simulink model "AttitudePlayground"  (R2024b)
settings: Solver=FixedStepAuto  StartTime=0.0  StopTime=inf  FixedStep=delta_t  RelTol=1e-3  EnableMultiTasking=on
values from neighbouring files (symbols this model uses):
  A = [eye(3), delta_t * eye(3) ... (first row only)    [AttitudePlayground_Vars.m]    (also in ParameterIdentification.m = [0 1)
  A_ESO = [1-l1_ESO, delta_t-l1_ESO*delta_t ... (first row only)    [AttitudePlayground_Vars.m]
  A_kalman = [1 delta_t ... (first row only)    [AttitudePlayground_Vars.m]    (also in ControlSystem_Vars.m)
  acc_sigma = 0.2 * calc_sigma(acc_pp)    [AttitudePlayground_Vars.m]    (also in ControlSystem_Vars.m)
  alpha_comp_pitch = calc_alpha(0.1, delta_t)    [AttitudePlayground_Vars.m]
  alpha_comp_roll = calc_alpha(0.1, delta_t)    [AttitudePlayground_Vars.m]
  alpha_comp_yaw = calc_alpha(1, delta_t)    [AttitudePlayground_Vars.m]
  B = zeros(6,3)    [AttitudePlayground_Vars.m]    (also in ParameterIdentification.m = [0)
  b_ESO = [b0_ESO*delta_t - l1_ESO*b0_ESO*delta_t ... (first row only)    [AttitudePlayground_Vars.m]
  bias_0 = [0, 0, 0]    [AttitudePlayground_Vars.m]
  bias_sigma = 0.000000001    (= 1e-09)    [AttitudePlayground_Vars.m]
  C = eye(6)    [AttitudePlayground_Vars.m]    (also in ParameterIdentification.m = [1 0])
  C_kalman = eye(2)    [AttitudePlayground_Vars.m]    (also in ControlSystem_Vars.m)
  delta_t = 0.01    [AttitudePlayground_Vars.m]    (also in ControlSystem_Vars.m; ParameterIdentification.m = t2 - t1)
  gyro_sigma = 1*((pi/180) * (0.07))    (= 0.0012217304764)    [AttitudePlayground_Vars.m]    (also in ControlSystem_Vars.m)
  gyro_sigma_3d = [1*gyro_sigma, 1*gyro_sigma, gyro_sigma]    [AttitudePlayground_Vars.m]    (also in ControlSystem_Vars.m)
  k_i_mahony = 0.0057    [AttitudePlayground_Vars.m]
  k_p_mahony = 0.42    [AttitudePlayground_Vars.m]
  l = [l1_ESO, l2_ESO]'    [AttitudePlayground_Vars.m]
  mag_sigma = 0.8 * calc_sigma(mag_pp)    [AttitudePlayground_Vars.m]
  P_0 = eye(4)    [AttitudePlayground_Vars.m]    (also in ControlSystem_Vars.m)
  P_0_gb = eye(7)    [AttitudePlayground_Vars.m]
  q_init = [cos(initial_yaw/2), 0, 0, sin(initial_yaw/2)]    [AttitudePlayground_Vars.m]
  q_sigma = 0.001    [AttitudePlayground_Vars.m]    (also in ControlSystem_Vars.m)
  R = 1.8 * diag([0.001396263^2, 0.0016580628^2, 0.05^2, ((pi/180) *              (0.05))^2, ((pi/180) * (0.07))^2, ((pi/180) * (0.07))^2])    [AttitudePlayground_Vars.m]    (also in ControlSystem_Vars.m = 0.015625)
  R_kalman = diag([(calc_sigma(0.8))^2, (0.07)^2])    [AttitudePlayground_Vars.m]    (also in ControlSystem_Vars.m)
  r_qekf = 1/sqrt(cos(magnetic_dip_angle_theta)^2 +      sin(magnetic_dip_angle_theta)^2)  * transpose([cos(magnetic_dip_angle_theta),0, sin(magnetic_dip_angle_theta)])    [AttitudePlayground_Vars.m]
  step_time = 10    [AttitudePlayground_Vars.m]
  tau_pitch_comp = 0.5    [AttitudePlayground_Vars.m]
  tau_roll_comp = 0.5    [AttitudePlayground_Vars.m]
  tau_yaw_comp = 3    [AttitudePlayground_Vars.m]
  Ts = delta_t    (= 0.01)    [AttitudePlayground_Vars.m]
  Ts2 = delta_t/2    (= 0.005)    [AttitudePlayground_Vars.m]
  Ts_IMU = delta_t    (= 0.01)    [AttitudePlayground_Vars.m]
  voltage_divider_Vout_max = 1.728    [AttitudePlayground_Vars.m]
undefined symbols (not defined in the file or in its folder): DiscIntNeverNeededParam, Discrete, Newton, Raphson, Time
libraries: simulink_extras x26, dspsigops x5, bbblueActuatorLib x4, ctrlSharedLib x2, matrix_library x2, dspmathops x2, dspstat3 x1, bbblueSensorLib x1, simulink x1, dspfdesign x1, bbblueBasicLib x1, vrlib x1
(part 1 of 3)
settings Model: ExtModeBatchMode=on  ExtModeTrigDuration=100  Creator=Henrik  LastModifiedBy=Henrik
settings SolverCC: PositivePriorityOrder=on
settings OptimizationCC: DefaultParameterBehavior=Inlined  EnhancedBackFolding=on  PassReuseOutputArgsAs=Individual arguments  ZeroExternalMemoryAtStartup=off  ZeroInternalMemoryAtStartup=off  MaxStackSize=64  OptimizeBlockOrder=speed  DifferentSizesBufferReuse=on  OptimizationCustomize=off  EfficientTunableParamExpr=on
settings DebuggingCC: ParameterTunabilityLossMsg=error
settings HardwareCC: ProdBitPerPointer=32  ProdBitPerSizeT=32  ProdBitPerPtrDiffT=32  ProdLargestAtomicInteger=Long  ProdLargestAtomicFloat=Double  ProdWordSize=32  ProdHWDeviceType=ARM Compatible->ARM Cortex-A (32-bit)  UseEmbeddedCoderFeatures=off
settings SFSimCC: MATLABDynamicMemAlloc=off
settings RTWCC: Description=Embedded Coder  SystemTargetFile=ert.tlc  HardwareBoard=BeagleBone Blue  TLCOptions="-aInlineSetEventsForThisBaseRateFcn=TLC_FALSE -aSuppressMultiTaskScheduler=TLC_FALSE  -aRateBasedStepFcn=0"  TemplateMakefile=ert_default_tmf  Toolchain=GNU GCC BeagleBone Blue
settings CodeAppCC: ForceParamTrailComments=on  IgnoreCustomStorageClasses=off  OperatorAnnotations=on  SimulinkDataObjDesc=on  SFDataObjDesc=on  InsertBlockDesc=on
settings ERTTargetCC: SupportNonInlinedSFcns=on  SupportVariableSizeSignals=on

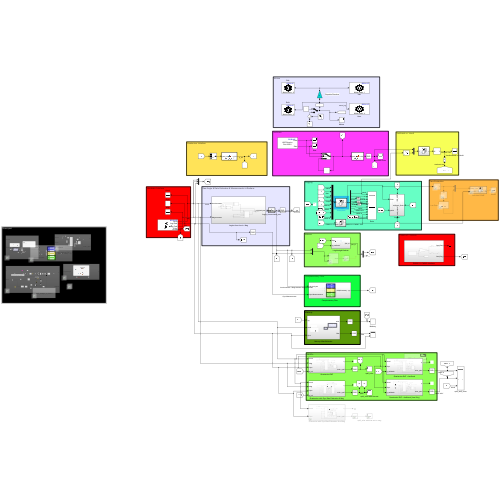
[thumbnail: Simulink's stored preview of the top-level diagram]
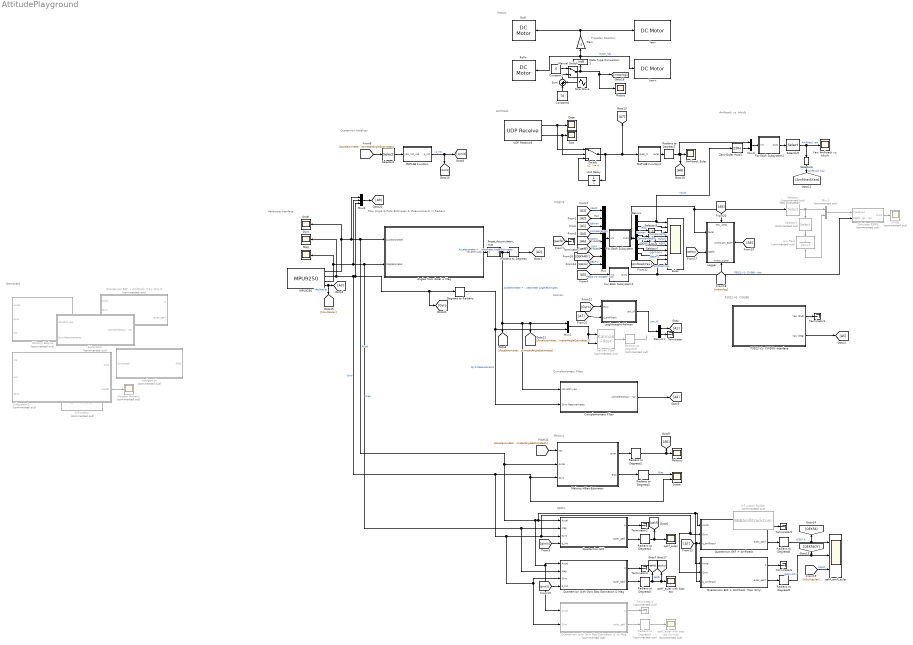
== system AttitudePlayground ==
  note: Graveyard
  note: Propeller Direction
  note: Motors
  note: Quaternion Initializer
  note: Amfitrack vs. Inbuilt
  note: Amfitrack
  note: QEKFs
  note: Mahony
  note: Yaw Evaluation
  note: P3022-V1- CW360
  note: Logging
  note: Kalman
  note: Raw Angle & Rate Estimates & Measurements in Radians
  note: Hardware Interface
  note: Complementary Filter
  Accel : Scope
  Amfitrack Euler : Scope
  Angle_Accumulator_mat : Subsystem  TreatAsAtomicUnit=on
  Angles from Accel + Mag : Subsystem
  Calculate RSME : Subsystem  Commented=on  TreatAsAtomicUnit=on
  Complementary Filter : Subsystem
  Constant1 : Constant  Value=0
  Constant2 : Constant  Value=70
  Data : Scope
  Data Type Conversion1 : DataTypeConversion  OutDataTypeStr=int8  SaturateOnIntegerOverflow=off  RndMeth=Floor
  Degrees to Radians : simulink_extras/Transformations/Degrees to Radians
  Demux : Demux  Outputs=8
  Demux1 : Demux  Outputs=2
  Euler : Scope  NumInputPorts=10
  For Each Subsystem : Subsystem  TreatAsAtomicUnit=on
  For Each Subsystem1 : Subsystem  TreatAsAtomicUnit=on
  For Each Subsystem2 : Subsystem  TreatAsAtomicUnit=on
  Gain : Gain  Gain=-1  OutDataTypeStr=int8
  Gyro : Scope
  Hossein Mahony : Scope  Commented=on
  Kalman Filter : ctrlSharedLib/Kalman Filter  Commented=on  TimeDomain=Discrete-Time  UseCurrentEstimator=on  ModelSource=Individual A, B, C, D matrices  ModelSourceVariable=ss(0.95,1,1,0,1)  A=A  B=B  C=C  D=0  NumberOfStates=1  NumberOfInputs=1  NumberOfOutputs=1  InitialEstimateSource=Input port  X0=0  P0=10  UseK=off  UseGH=off  NumberOfProcessNoiseInputs=1  G=1  TimeInvariantG=on  H=0  TimeInvariantH=on  Q=Q  TimeInvariantQ=on  R=R  TimeInvariantR=on  N=0  TimeInvariantN=on  AddInputPort=off  AddEnablePort=off  OutputEstimatedY=off  OutputP=off  Ts=delta_t
  Leightweight-Kalman : Subsystem
  Logger : Subsystem
      settings: PortSchema="{\"entries\":[{\"content\":{\"sides\":[{\"content\":{\"connectorIds\":[\"In1\",\"In2\"]},\"type\":\"ConnectorPlacement.EquallySpacedRectSide\",\"uuid\":\"65dae65f-b2e3-411c-80c9-991e84581ea0\"},{\"content\":{\"connectorIds\":[\"In5\"],\"side\":\"RIGHT\"},\"type\":\"ConnectorPlacement.EquallySpacedRectSide\",\"uuid\":\"096d2477-2900-49bd-8ed4-d95fcaab5e6a\"},{\"content\":{\"connectorIds\":[\"In3\"],\"side\":\"TOP\"},\"type\":\"ConnectorPlacement.EquallySpacedRectSide\",\"uuid\":\"63021306-1025-463e-9144-c93885efa2cd\"},{\"content\":{\"connectorIds\":[\"In4\"],\"side\":\"BOTTOM\"},\"type\":\"ConnectorPlacement.EquallySpacedRectSide\",\"uuid\":\"f0130dd7-b4e5-4c0e-a86a-26aff2d064e3\"}]},\"type\":\"ConnectorPlacement.EquallySpacedConnector\",\"uuid\":\"57989227-06af-4d59-a161-01dcfc1f7af4\"}],\"packageUris\":[\"http://schema.mathworks.com/mf0/Connector/R2020b\"],\"version\":\"1.0\"}"
  Low Pass : TransferFcn  Commented=on  Denominator=[10 1]
  MATLAB Function : MATLAB Function  TreatAsAtomicUnit=on
  MATLAB Function1 : MATLAB Function  TreatAsAtomicUnit=on
  MPU9250 : bbblueSensorLib/MPU9250  OperationMode=DMP  Accel=on  AngularRate=on  Ak8963Field=on  EulerAngles=on  Quat=off  AccelRange=2G  Acceldlpf=1  GyroRange=250 dps  Gyrodlpf=1  DmpOdr=200 Hz  SampleTime=delta_t
  Mag : Scope
  Mahony : Scope
  Mahony Backup : Subsystem  Commented=on
  Mahony+Bias-Estimator : Subsystem
  Manual Switch : ManualSwitch
  Motors : Scope
  Mux : Mux  Inputs=8
  Mux1 : Mux  Inputs=2
  Mux2 : Mux  Commented=on  Inputs=2
  Mux3 : Mux  Inputs=2
  Mux4 : Mux  Inputs=3
  P3022-V1- CW360 -Interface : Subsystem
  Quarternion EKF : Subsystem
  Quarternion EKF + Amfitrack : Subsystem
  Quarternion EKF + Amfitrack (Yaw Only) : Subsystem
  Quarternion EKF + Amfitrack (Yaw Only)1 : Subsystem  Commented=on
  Quarternion with Gyro Bias Estimation & Mag : Subsystem
  Quarternion with Gyro Bias Estimation & no Mag : Subsystem  Commented=on
  RMSE : Scope  Commented=on
  Radians to Degrees{,2..5,7..9} (8 alike) : simulink_extras/Transformations/Radians to Degrees
  Radians to Degrees1 : simulink_extras/Transformations/Radians to Degrees  Commented=on
  Radians to Degrees6 : simulink_extras/Transformations/Radians to Degrees  Commented=on
  Roll+ : bbblueActuatorLib/DC Motor  index=3  stopaction=Free Spin  SimulateUsing=Code generation
  Roll- : bbblueActuatorLib/DC Motor  index=2  stopaction=Free Spin  SimulateUsing=Code generation
  S-Function : S-Function  Commented=on  FunctionName=amfi_beagle_s_func.c  SFunctionDeploymentMode=off  EnableBusSupport=off
  S-Function Builder : S-Function  Commented=on  FunctionName=BBBAmflitrackCom  SFunctionModules=BBBAmflitrackCom_wrapper.cpp  SFunctionDeploymentMode=off  EnableBusSupport=off  mask(S-Function Builder){}
      mask help: Simulink:masks:SFunctionBuilder_MD
      mask init:
      | val = [[.9  0.75 0.75 1 1 .9 .9 1]',[1 1 0.75 0.75 .9 .9 1 .9]'];try , sys = get_param(gcb,'SfunBuilderFcnName');if isempty(sys), sys = get_param(gcb,'FunctionName'); end,catch, sys = get_param(gcb,'FunctionName'); end
      settings: CopyFcn=set_param(gcbh,'LinkStatus','none')  OpenFcn=sfunctionwizard(gcbh)
      mask Display:
      | plot(val(:,1),val(:,2))
      | disp(sys)
      | port_label('input',1,sprintf('%s', 'u0'),'interpreter','tex')
      | port_label('output',1,sprintf('%s', 'y0'),'interpreter','tex')
  Scope : Scope  NumInputPorts=2
  Selector : Selector  Commented=on  InputPortWidth=24  IndexOptions=Index vector (dialog)  Indices=[3 6 9 12 15 18 21 24]  OutputSizes=1
  Selector1 : Selector  Commented=on  InputPortWidth=8  IndexOptions=Index vector (dialog)  Indices=[2]  OutputSizes=1
  Selector2 : Selector  InputPortWidth=3  IndexOptions=Index vector (dialog)  Indices=[ 3]  OutputSizes=1
  Selector3 : Selector  InputPortWidth=3  IndexOptions=Index vector (dialog)  Indices=[3]  OutputSizes=1
  Selector4 : Selector  InputPortWidth=3  IndexOptions=Index vector (dialog)  Indices=[3]  OutputSizes=1
  Selector5 : Selector  InputPortWidth=6  IndexOptions=Index vector (dialog)  Indices=[3 6]  OutputSizes=1
  Selector6 : Selector  InputPortWidth=2  IndexOptions=Index vector (dialog)  Indices=[1]  OutputSizes=1
  Selector7 : Selector  InputPortWidth=3  IndexOptions=Index vector (dialog)  Indices=[3]  OutputSizes=1
  Sine Wave : Sin  Amplitude=15  Frequency=0.05*(2*pi)  SampleTime=delta_t
  Size : Scope
  Subsystem : Subsystem  Commented=on
  Subsystem3 : Subsystem  Commented=on
  Sum : Sum  Inputs=|++
  Switch : Switch  Threshold=4  SaturateOnIntegerOverflow=off  InputSameDT=off
  Terminator{,1..3,5..7} (7 alike) : Terminator
  Terminator4 : Terminator  Commented=on
  UDP Receive5 : bbblueCommlib/UDP Receive  localURL='0.0.0.0'  localPort=25001  remoteURL='0.0.0.0'  remotePort=-1  recvBufferSize=8192  signalDatatype=double  dims=4  isVarSize=off  showBlockingTime=off  blockingTime=0  sampletime=0.01  blockPlatform=BB BLUE
  Unit Delay : UnitDelay  InitialCondition=[1,0,0,0]'  SampleTime=-1  HasFrameUpgradeWarning=on
  Yaw Amfitrack vs. Inbuilt : Scope
  Yaw+ : bbblueActuatorLib/DC Motor  index=4  stopaction=Free Spin  SimulateUsing=Code generation
  Yaw- : bbblueActuatorLib/DC Motor  index=1  stopaction=Free Spin  SimulateUsing=Code generation
  Zero-Order Hold1 : ZeroOrderHold  SampleTime=0.01
  madgewick : Subsystem  Commented=on
  qekf_amfi_euler : Scope  NumInputPorts=3
  qekf_euler : Scope
  qekf_euler with bias est : Scope
  qekf_euler with bias est no mag : Scope  Commented=on
  wires:
  MPU9250/1 -> Mux4/1, Quarternion with Gyro Bias Estimation & no Mag/1(Accel), Quarternion with Gyro Bias Estimation & Mag/1(Accel), Quarternion EKF/1(Accel), Quarternion EKF + Amfitrack (Yaw Only)/1(Accel), Quarternion EKF + Amfitrack/1(Accel), Mahony+Bias-Estimator/2(Accel), Angles from Accel + Mag/1(Accelerometer), Accel/1  "Accel"
  MPU9250/2 -> Mux4/3, Degrees to Radians/1, [Gyro], Quarternion with Gyro Bias Estimation & no Mag/2(Gyro), Quarternion with Gyro Bias Estimation & Mag/3(Gyro), Quarternion EKF/3(Gyro), Quarternion EKF + Amfitrack (Yaw Only)/2(Gyro), Quarternion EKF + Amfitrack/2(Gyro), Scope/2, Mahony+Bias-Estimator/3(Gyro), Gyro/1  "Gyro"
  MPU9250/3 -> Mux4/2, Quarternion with Gyro Bias Estimation & Mag/2(Mag), Quarternion EKF/2(Mag), Angles from Accel + Mag/2(Magnetometer), Mag/1  "mag"
  Angle_Accumulator_mat/1(angle_acc) -> [AccelerometerMagnetometerAngleEstimates], [AccelerometerMagnetometerAngleEstimates1], Mux1/1, Complementary Filter/1(roll,pitch,yaw), Radians to Degrees/1  "Accelerometer + Magnetometer Angle Estimates"
  Mux1/1 -> Kalman Filter/2, Kalman Filter/1
  Radians to Degrees1/1 -> ?
  Demux1/2 -> Terminator/1
  Kalman Filter/1 -> Radians to Degrees1/1
  Demux1/1 -> [A1]
  Demux/3 -> Selector3/1  "Kalman"
  Radians to Degrees/1 -> [A2]
  Demux/2 -> Euler/2  "Raw"
  MPU9250/4 -> [inbuilteuler], [A3]  "inbuilteuler"
  Demux/1 -> Zero-Order Hold1/1, Euler/1  "Inbuilt"
  Degrees to Radians/1 -> Complementary Filter/2(Gyro Measurements), Mux1/2  "Gyro Measurements"
  Complementary Filter/1(complementary - rpy) -> [A4]
  Demux/4 -> Selector4/1  "Complementary"
  P3022-V1- CW360 -Interface/1(Yaw (Rad)) -> Terminator1/1
  P3022-V1- CW360 -Interface/2(Yaw (Deg)) -> [A5]
  For Each Subsystem1/1(Out1) -> Calculate RSME/2(P3022-V1- CW360 - Yaw), Euler/9  "P3022-V1- CW360 - Yaw"
  [A3] -> Mux/1  "Inbuilt"
  [A2] -> Mux/2  "Raw"
  [A1] -> Mux/3  "Kalman"
  [A4] -> Mux/4  "Complementary"
  [A5] -> For Each Subsystem1/1(In1)  "P3022-V1- CW360 - Yaw"
  Mux/1 -> For Each Subsystem/1(In1)
  For Each Subsystem/1(Out1) -> Logger/1(Euler), Selector/1, Demux/1
  Mahony+Bias-Estimator/1(euler) -> Radians to Degrees2/1
  Radians to Degrees2/1 -> [A6], Mahony/1
  Selector/1 -> Mux2/1, Selector1/1
  Calculate RSME/1(Out1) -> RMSE/1
  Selector1/1 -> Low Pass/1
  Low Pass/1 -> Mux2/2
  Mux2/1 -> Calculate RSME/1(Fused Yaw)
  Subsystem3/2(Angles) -> Hossein Mahony/1
  [A6] -> Mux/5  "Mahony"
  Selector7/1 -> Euler/5  "Mahony"
  Mahony+Bias-Estimator/2(Bias) -> Radians to Degrees3/1
  Radians to Degrees3/1 -> Scope/1  "Bias"
  Quarternion EKF/2(euler_qekf) -> Radians to Degrees4/1
  Quarternion EKF/1(q) -> Terminator2/1
  Radians to Degrees4/1 -> [qekf], qekf_euler/1
  [qekf] -> Mux/6  "QEKF"
  Demux/6 -> Euler/6  "QEKF"
  Radians to Degrees5/1 -> [qekfb1], qekf_euler with bias est/1, [qekfb]  "qekfb"
  Quarternion with Gyro Bias Estimation & Mag/1(q) -> Terminator3/1
  Quarternion with Gyro Bias Estimation & Mag/2(euler_qekf) -> Radians to Degrees5/1
  Quarternion with Gyro Bias Estimation & no Mag/1(q) -> Terminator4/1
  Quarternion with Gyro Bias Estimation & no Mag/2(euler_qekf) -> Radians to Degrees6/1
  Radians to Degrees6/1 -> qekf_euler with bias est no mag/1
  Demux/7 -> Euler/7  "QEKF-AOY"
  Selector2/1 -> MATLAB Function/1(yaw_init_rad)
  [AccelerometerMagnetometerAngleEstimates] -> Selector2/1
  MATLAB Function/1(q_init) -> [qinit1], [qinit]  "q_init"
  [qinit] -> Quarternion EKF/4(q_init)
  [qinit1] -> Quarternion with Gyro Bias Estimation & Mag/4(q_init)
  Selector3/1 -> Euler/3  "Kalman"
  Selector4/1 -> Euler/4  "Complementary"
  Radians to Degrees7/1 -> [A8], Amfitrack Euler/1, Mux3/1
  Unit Delay/1 -> Switch/3
  MATLAB Function1/1(euler) -> Radians to Degrees7/1
  UDP Receive5/2 -> Switch/2, Size/1
  UDP Receive5/1 -> Switch/1, Data/1
  Mux3/1 -> For Each Subsystem2/1(In1)
  For Each Subsystem2/1(Out1) -> Selector5/1
  Zero-Order Hold1/1 -> Mux3/2
  [AccelerometerMagnetometerAngleEstimates1] -> Mahony+Bias-Estimator/1(rpy)
  Selector5/1 -> Selector6/1, Yaw Amfitrack vs. Inbuilt/1  "Amfitrack Yaw"
  Selector6/1 -> [AmfitrackYaw]  "Amfitrack Yaw"
  [AmfitrackYaw] -> Euler/10  "AmfitrackYaw"
  Angles from Accel + Mag/1(roll,pitch,yaw) -> Angle_Accumulator_mat/1(angle)  "Accelerometer + Magnetometer Angle Estimates"
  [A7] -> Quarternion EKF + Amfitrack (Yaw Only)/3(q_amfitrack), Quarternion EKF + Amfitrack/3(q_amfitrack)
  Quarternion EKF + Amfitrack/2(euler_qekf) -> Radians to Degrees8/1
  Radians to Degrees8/1 -> [QEKFA], qekf_amfi_euler/1  "QEKF-A"
  Quarternion EKF + Amfitrack/1(q) -> Terminator5/1
  Demux/8 -> Euler/8  "QEKF-A"
  [QEKFA] -> Mux/8  "QEKF-A"
  Sum/1 -> Manual Switch/2
  Gain/1 -> Yaw-/1, Roll-/1
  Data Type Conversion1/1 -> Yaw+/1, Roll+/1, Gain/1  "motor_log"
  Quarternion EKF + Amfitrack (Yaw Only)/2(euler_qekf) -> Radians to Degrees9/1
  Quarternion EKF + Amfitrack (Yaw Only)/1(q) -> Terminator6/1
  Radians to Degrees9/1 -> [QEKFAOY], qekf_amfi_euler/2  "QEKF-AOY"
  [inbuilteuler] -> qekf_amfi_euler/3  "Inbuilt"
  Demux/5 -> Selector7/1  "Mahony"
  [qekfb] -> Terminator7/1
  [QEKFAOY] -> Mux/7
  Switch/1 -> [A7], MATLAB Function1/1(quat_in), Unit Delay/1
  [qekfb1] -> Logger/2(qekfb)
  [motorlog] -> Logger/4(motor_signal)
  [A8] -> Logger/5(Amfitrack_Euler)
  Mux4/1 -> [A9]
  [A9] -> Logger/3(IMU_AMG)
  Constant2/1 -> Sum/1
  Sine Wave/1 -> Sum/2
  Constant1/1 -> Manual Switch/1
  Manual Switch/1 -> Motors/1, [motorlog], Data Type Conversion1/1
  [A7] -> Leightweight-Kalman/2(q_amfitrack)
  Leightweight-Kalman/1(yaw_kf) -> Demux1/1  "yaw_kf"
  [Gyro] -> Leightweight-Kalman/1(Gyro)

== system AttitudePlayground/Angle_Accumulator_mat ==
  angle : Inport  Partition=on  PartitionDimension=1  PartitionWidth=1  PartitionOffset=0
  Angle accumulator : Subsystem
  Degrees to Radians : simulink_extras/Transformations/Degrees to Radians
  For Each : ForEach  DisableCoverage=on
  Radians to Degrees : simulink_extras/Transformations/Radians to Degrees
  angle_acc : Outport  ConcatenationDimension=1
  wires:
  angle/1 -> Radians to Degrees/1
  Angle accumulator/1(angle_acc) -> Degrees to Radians/1
  Radians to Degrees/1 -> Angle accumulator/1(angle)
  Degrees to Radians/1 -> angle_acc/1

== system AttitudePlayground/Angles from Accel + Mag ==
  Accelerometer : Inport
  Magnetometer : Inport  Port=2
  Demux : Demux  Outputs=3
  Demux2 : Demux  Outputs=3
  MATLAB Function : MATLAB Function  TreatAsAtomicUnit=on
  MATLAB Function1 : MATLAB Function  TreatAsAtomicUnit=on
  MATLAB Function2 : MATLAB Function  TreatAsAtomicUnit=on
  Mux : Mux  Inputs=3
  roll,pitch,yaw : Outport
  wires:
  Accelerometer/1 -> Demux/1
  Demux/1 -> MATLAB Function1/1(a_x)
  Demux/3 -> MATLAB Function1/3(a_z), MATLAB Function/2(a_z)  "az"
  Demux/2 -> MATLAB Function1/2(a_y), MATLAB Function/1(a_y)  "ay"
  Magnetometer/1 -> Demux2/1
  MATLAB Function/1(roll) -> MATLAB Function1/4(roll), Mux/1, MATLAB Function2/1(roll)  "roll"
  MATLAB Function1/1(pitch) -> Mux/2, MATLAB Function2/2(pitch)  "pitch"
  Demux2/1 -> MATLAB Function2/3(m_x)
  Demux2/2 -> MATLAB Function2/4(m_y)
  Demux2/3 -> MATLAB Function2/5(m_z)
  Mux/1 -> roll,pitch,yaw/1
  MATLAB Function2/1(yaw) -> Mux/3  "yaw"

== system AttitudePlayground/Calculate RSME ==
  Fused Yaw : Inport  Partition=on  PartitionDimension=1  PartitionWidth=1  PartitionOffset=0
  P3022-V1- CW360 - Yaw : Inport  Port=2
  For Each : ForEach  DisableCoverage=on
  RMS1 : dspstat3/RMS  run=on  directionMode=Each column  dimension=1  reset_popup=Rising edge
  Reset : Subsystem  TreatAsAtomicUnit=on
  Step : Step  Time=step_time  SampleTime=0
  Sum : Sum  Inputs=|+-
  Zero-Order Hold : ZeroOrderHold  SampleTime=delta_t
  Zero-Order Hold1 : ZeroOrderHold  SampleTime=delta_t
  Out1 : Outport  ConcatenationDimension=1
  wires:
  Sum/1 -> Zero-Order Hold/1
  Fused Yaw/1 -> Sum/1
  P3022-V1- CW360 - Yaw/1 -> Sum/2
  Reset/1(Out1) -> Out1/1
  RMS1/1 -> Reset/1(In1)
  Zero-Order Hold/1 -> RMS1/1
  Step/1 -> Zero-Order Hold1/1
  Zero-Order Hold1/1 -> RMS1/2

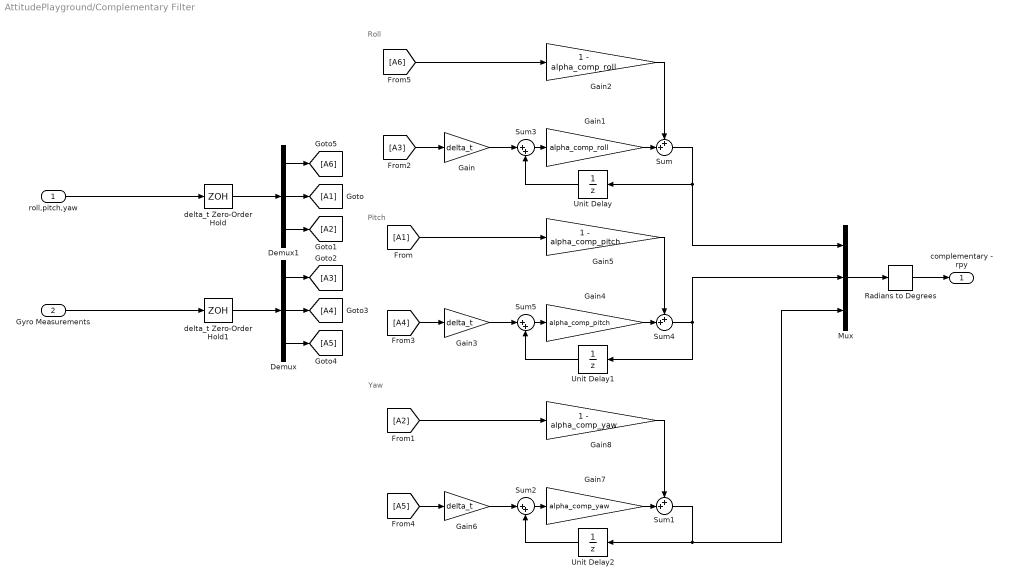
== system AttitudePlayground/Complementary Filter ==
  note: Yaw
  note: Pitch
  note: Roll
  roll,pitch,yaw : Inport
  Gyro Measurements : Inport  Port=2
  Demux : Demux  Outputs=3
  Demux1 : Demux  Outputs=3
  Gain : Gain  Gain=delta_t
  Gain1 : Gain  Gain=alpha_comp_roll
  Gain2 : Gain  Gain=1 - alpha_comp_roll
  Gain3 : Gain  Gain=delta_t
  Gain4 : Gain  Gain=alpha_comp_pitch
  Gain5 : Gain  Gain=1 - alpha_comp_pitch
  Gain6 : Gain  Gain=delta_t
  Gain7 : Gain  Gain=alpha_comp_yaw
  Gain8 : Gain  Gain=1 - alpha_comp_yaw
  Mux : Mux  Inputs=3
  Radians to Degrees : simulink_extras/Transformations/Radians to Degrees
  Sum : Sum  Inputs=++|
  Sum1 : Sum  Inputs=++|
  Sum2 : Sum  Inputs=|++
  Sum3 : Sum  Inputs=|++
  Sum4 : Sum  Inputs=++|
  Sum5 : Sum  Inputs=|++
  Unit Delay : UnitDelay  SampleTime=delta_t  HasFrameUpgradeWarning=on
  Unit Delay1 : UnitDelay  SampleTime=delta_t  HasFrameUpgradeWarning=on
  Unit Delay2 : UnitDelay  SampleTime=delta_t  HasFrameUpgradeWarning=on
  delta_t Zero-Order Hold : ZeroOrderHold  SampleTime=delta_t
  delta_t Zero-Order Hold1 : ZeroOrderHold  SampleTime=delta_t
  complementary - rpy : Outport
  wires:
  Gyro Measurements/1 -> delta_t Zero-Order Hold1/1
  roll,pitch,yaw/1 -> delta_t Zero-Order Hold/1
  Mux/1 -> Radians to Degrees/1
  Radians to Degrees/1 -> complementary - rpy/1
  Demux1/2 -> [A1]
  Demux1/3 -> [A2]
  Demux/1 -> [A3]
  [A3] -> Gain/1
  Demux/2 -> [A4]
  Demux/3 -> [A5]
  Demux1/1 -> [A6]
  [A6] -> Gain2/1
  delta_t Zero-Order Hold/1 -> Demux1/1
  delta_t Zero-Order Hold1/1 -> Demux/1
  Gain/1 -> Sum3/1
  Sum3/1 -> Gain1/1
  Gain1/1 -> Sum/2
  Gain2/1 -> Sum/1
  Sum/1 -> Mux/1, Unit Delay/1
  Unit Delay/1 -> Sum3/2
  Gain3/1 -> Sum5/1
  Gain5/1 -> Sum4/1
  Unit Delay1/1 -> Sum5/2
  Sum5/1 -> Gain4/1
  [A1] -> Gain5/1
  [A4] -> Gain3/1
  Sum4/1 -> Unit Delay1/1, Mux/2
  Gain4/1 -> Sum4/2
  Gain6/1 -> Sum2/1
  Gain8/1 -> Sum1/1
  Unit Delay2/1 -> Sum2/2
  Sum2/1 -> Gain7/1
  [A2] -> Gain8/1
  [A5] -> Gain6/1
  Sum1/1 -> Mux/3, Unit Delay2/1
  Gain7/1 -> Sum1/2

== system AttitudePlayground/For Each Subsystem ==
  In1 : Inport  Partition=on  PartitionDimension=1  PartitionWidth=1  PartitionOffset=0
  For Each : ForEach  DisableCoverage=on
  Sample and Hold : dspsigops/Sample and Hold  trig=Rising edge  initCond=0  latchinput=off
  Step : Step  Time=step_time  SampleTime=0
  Sum : Sum  Inputs=|+-
  Yaw accumulator : Subsystem
  Out1 : Outport  SampleTime=delta_t  ConcatenationDimension=1
  wires:
  Yaw accumulator/1(yaw_acc) -> Sum/1, Sample and Hold/1
  Sample and Hold/1 -> Sum/2
  Step/1 -> Sample and Hold/Trigger
  Sum/1 -> Out1/1
  In1/1 -> Yaw accumulator/1(yaw)

== system AttitudePlayground/For Each Subsystem1 ==
  In1 : Inport  SampleTime=delta_t  Partition=on  PartitionDimension=1  PartitionWidth=1  PartitionOffset=0
  For Each : ForEach  DisableCoverage=on
  Sample and Hold : dspsigops/Sample and Hold  trig=Rising edge  initCond=0  latchinput=off
  Step : Step  Time=step_time  SampleTime=delta_t
  Sum : Sum  Inputs=|+-
  Out1 : Outport  ConcatenationDimension=1
  wires:
  In1/1 -> Sum/1, Sample and Hold/1
  Sample and Hold/1 -> Sum/2
  Step/1 -> Sample and Hold/Trigger
  Sum/1 -> Out1/1

== system AttitudePlayground/For Each Subsystem2 ==
  In1 : Inport  Partition=on  PartitionDimension=1  PartitionWidth=1  PartitionOffset=0
  For Each : ForEach  DisableCoverage=on
  Sample and Hold : dspsigops/Sample and Hold  trig=Rising edge  initCond=0  latchinput=off
  Step : Step  Time=step_time  SampleTime=0.01
  Sum : Sum  Inputs=|+-
  Yaw accumulator : Subsystem
  Out1 : Outport  ConcatenationDimension=1
  wires:
  Yaw accumulator/1(yaw_acc) -> Sample and Hold/1, Sum/1
  Sample and Hold/1 -> Sum/2
  Step/1 -> Sample and Hold/Trigger
  Sum/1 -> Out1/1
  In1/1 -> Yaw accumulator/1(yaw)

== system AttitudePlayground/Leightweight-Kalman ==
  Gyro : Inport
  q_amfitrack : Inport  Port=2
  Constant : Constant  Value=0
  Demux : Demux  Outputs=2
  Initialize KF : MATLAB Function  TreatAsAtomicUnit=on
  Kalman Filter : ctrlSharedLib/Kalman Filter  TimeDomain=Discrete-Time  UseCurrentEstimator=on  ModelSource=Individual A, B, C, D matrices  ModelSourceVariable=ss(0.95,1,1,0,1)  A=A_kalman  B=1  C=C_kalman  D=0  NumberOfStates=1  NumberOfInputs=1  NumberOfOutputs=1  InitialEstimateSource=Input port  X0=0  P0=10  UseK=off  UseGH=off  NumberOfProcessNoiseInputs=1  G=1  TimeInvariantG=on  H=0  TimeInvariantH=on  Q=Q_kalman  TimeInvariantQ=on  R=R_kalman  TimeInvariantR=on  N=0  TimeInvariantN=on  AddInputPort=off  AddEnablePort=off  OutputEstimatedY=off  OutputP=off  Ts=-1
  MATLAB Function1 : MATLAB Function  TreatAsAtomicUnit=on
  MATLAB Function2 : MATLAB Function  TreatAsAtomicUnit=on
  Mux : Mux  Inputs=2
  Mux1 : Mux  Inputs=2
  Mux2 : Mux  Inputs=3
  Radians to Degrees1 : simulink_extras/Transformations/Radians to Degrees
  Radians to Degrees7 : simulink_extras/Transformations/Radians to Degrees
  Selector : Selector  InputPortWidth=3  IndexOptions=Index vector (dialog)  Indices=[3]  OutputSizes=1
  Selector1 : Selector  InputPortWidth=3  IndexOptions=Index vector (dialog)  Indices=[3]  OutputSizes=1
  Selector2 : Selector  InputPortWidth=3  IndexOptions=Index vector (dialog)  Indices=[3]  OutputSizes=1
  Terminator : Terminator
  Yaw accumulator1 : Subsystem
  yaw_kf : Outport
  wires:
  Gyro/1 -> Selector2/1  "original"
  q_amfitrack/1 -> MATLAB Function1/1(quat_in), Initialize KF/1(quat_meas)
  Initialize KF/1(q_init) -> MATLAB Function2/1(quat_in)  "q_init"
  Radians to Degrees7/1 -> Selector/1  "Amfitrack Euler"
  MATLAB Function1/1(euler) -> Radians to Degrees7/1
  MATLAB Function2/1(euler) -> Radians to Degrees1/1
  Radians to Degrees1/1 -> Selector1/1  "Amfitrack Euler"
  Selector1/1 -> Mux/1
  Mux/1 -> Kalman Filter/2
  Kalman Filter/1 -> Demux/1
  Selector/1 -> Yaw accumulator1/1(yaw)
  Mux1/1 -> Kalman Filter/1
  Yaw accumulator1/1(yaw_acc) -> Mux1/1
  Selector2/1 -> Mux1/2, Mux/2
  Mux2/1 -> yaw_kf/1
  Constant/1 -> Mux2/2, Mux2/1
  Demux/1 -> Mux2/3
  Demux/2 -> Terminator/1

== system AttitudePlayground/Logger ==
  Euler : Inport
  qekfb : Inport  Port=2
  IMU_AMG : Inport  Port=3
  motor_signal : Inport  Port=4
  Amfitrack_Euler : Inport  Port=5
  Demux : Demux  Outputs=8
  To File : ToFile  Filename=HENRIK_LOG_INBUILT.mat  MatrixName=INBUILT
  To File1 : ToFile  Filename=HENRIK_LOG_RAW.mat  MatrixName=RAW
  To File10 : ToFile  Filename=HENRIK_LOG_AMFITRACK_EULER.mat  MatrixName=AMFITRACK_EULER
  To File11 : ToFile  Filename=HENRIK_LOG_IMU_AMG.mat  MatrixName=IMU_AMG
  To File2 : ToFile  Filename=HENRIK_LOG_KALMAN.mat  MatrixName=KALMAN
  To File3 : ToFile  Filename=HENRIK_LOG_COMPLENTARY.mat  MatrixName=COMPLENTARY
  To File4 : ToFile  Filename=HENRIK_LOG_MAHONY.mat  MatrixName=MAHONY
  To File5 : ToFile  Filename=HENRIK_LOG_QEKF.mat  MatrixName=QEKF
  To File6 : ToFile  Filename=HENRIK_LOG_QEKF_AOY.mat  MatrixName=QEKF_AOY
  To File7 : ToFile  Filename=HENRIK_LOG_QEKF_A.mat  MatrixName=QEKF_A
  To File8 : ToFile  Filename=HENRIK_LOG_QEKF_B.mat  MatrixName=QEKF_B
  To File9 : ToFile  Filename=HENRIK_LOG_MOTOR_SIGNAL.mat  MatrixName=MOTOR_SIGNAL
  wires:
  Euler/1 -> Demux/1
  Demux/1 -> To File/1  "inbuilt"
  Demux/2 -> To File1/1  "raw"
  Demux/3 -> To File2/1  "kalman"
  Demux/4 -> To File3/1  "complementary"
  Demux/5 -> To File4/1  "Mahony"
  Demux/6 -> To File5/1  "qekf"
  Demux/7 -> To File6/1  "qekf-aoy"
  Demux/8 -> To File7/1  "qekf-a"
  qekfb/1 -> To File8/1  "qekf-b"
  motor_signal/1 -> To File9/1  "Motor Signal"
  Amfitrack_Euler/1 -> To File10/1  "Amfitrack_Euler"
  IMU_AMG/1 -> To File11/1  "ACCEL, MAG, GYRO"

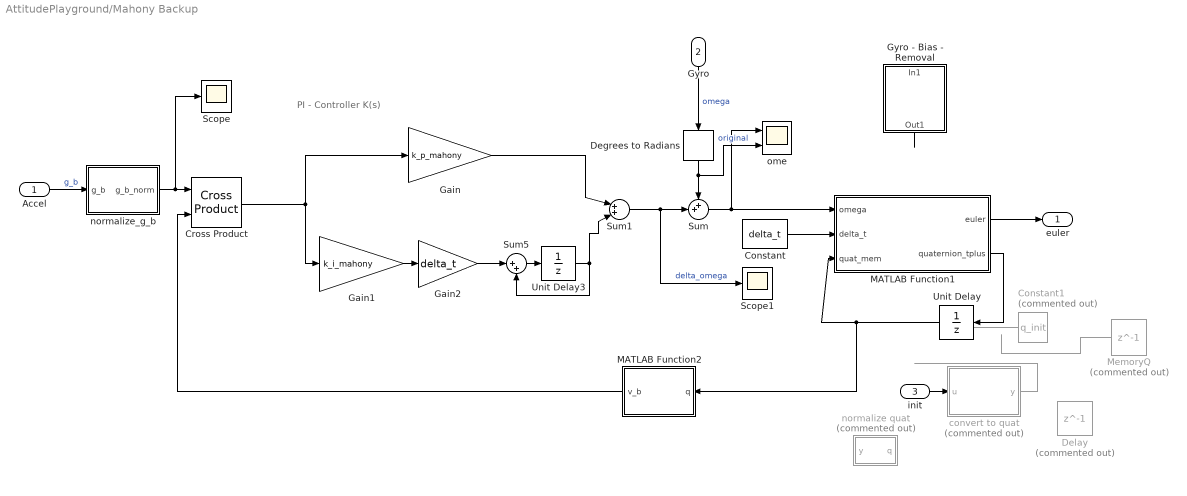
== system AttitudePlayground/Mahony Backup ==
  note: PI - Controller K(s)
  Accel : Inport
  Gyro : Inport  Port=2
  init : Inport  Port=3
  Constant : Constant  Value=delta_t
  Constant1 : Constant  Commented=on  Value=q_init  SampleTime=delta_t
  Cross Product : matrix_library/Cross Product
  Degrees to Radians : simulink_extras/Transformations/Degrees to Radians
  Delay : Delay  Commented=on  DelayLength=1  InitialConditionSource=Input port  SampleTime=delta_t
      settings: InputPortMap=u0,p4
  Gain : Gain  Gain=k_p_mahony
  Gain1 : Gain  Gain=k_i_mahony
  Gain2 : Gain  Gain=delta_t
  Gyro - Bias - Removal : Subsystem
  MATLAB Function1 : MATLAB Function  TreatAsAtomicUnit=on  SystemSampleTime=delta_t
  MATLAB Function2 : MATLAB Function  TreatAsAtomicUnit=on
  MemoryQ : Delay  Commented=on  DelayLength=1  InitialConditionSource=Input port  SampleTime=delta_t
      settings: InputPortMap=u0,p4
  Scope : Scope
  Scope1 : Scope
  Sum : Sum  Inputs=++|
  Sum1 : Sum  Inputs=|++|
  Sum5 : Sum  Inputs=|++
  Unit Delay : UnitDelay  InitialCondition=q_init  SampleTime=delta_t  HasFrameUpgradeWarning=on
  Unit Delay3 : UnitDelay  SampleTime=delta_t  HasFrameUpgradeWarning=on
  convert to quat : MATLAB Function  Commented=on  TreatAsAtomicUnit=on
  normalize quat : MATLAB Function  Commented=on  TreatAsAtomicUnit=on
  normalize_g_b : MATLAB Function  TreatAsAtomicUnit=on
  ome : Scope  NumInputPorts=2
  euler : Outport
  wires:
  MATLAB Function1/1(euler) -> euler/1
  Accel/1 -> normalize_g_b/1(g_b)  "g_b"
  Gyro/1 -> Degrees to Radians/1  "omega"
  Sum1/1 -> Scope1/1, Sum/2  "delta_omega"
  Constant/1 -> MATLAB Function1/2(delta_t)
  Degrees to Radians/1 -> ome/2, Sum/1  "original"
  MATLAB Function2/1(v_b) -> Cross Product/2
  Gain/1 -> Sum1/1
  Gain1/1 -> Gain2/1
  Cross Product/1 -> Gain1/1, Gain/1
  Unit Delay3/1 -> Sum1/2, Sum5/2
  Sum/1 -> ome/1, MATLAB Function1/1(omega)
  normalize_g_b/1(g_b_norm) -> Cross Product/1, Scope/1
  Unit Delay/1 -> MATLAB Function2/1(q), MATLAB Function1/3(quat_mem)
  Constant1/1 -> ?
  MATLAB Function1/2(quaternion_tplus) -> Unit Delay/1
  Gain2/1 -> Sum5/1
  Sum5/1 -> Unit Delay3/1
  init/1 -> convert to quat/1(u)
  MemoryQ/1 -> ?
  convert to quat/1(y) -> ?
  Gyro - Bias - Removal/1(Out1) -> ?
  ? -> Gyro - Bias - Removal/1(In1)

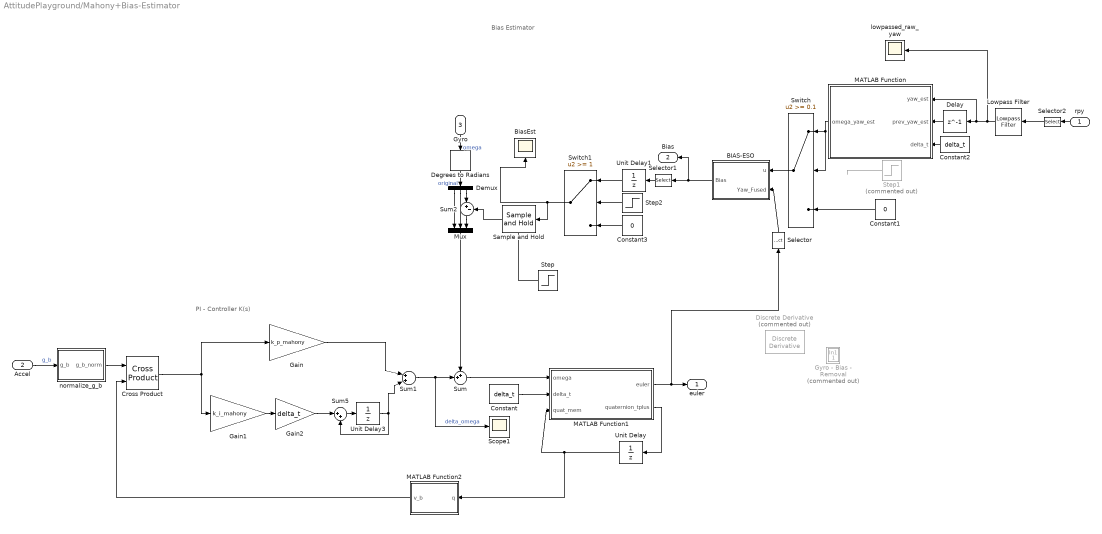
== system AttitudePlayground/Mahony+Bias-Estimator ==
  note: Bias Estimator
  note: PI - Controller K(s)
  rpy : Inport
  Accel : Inport  Port=2
  Gyro : Inport  Port=3
  BIAS-ESO : Subsystem
  BiasEst : Scope
  Constant : Constant  Value=delta_t
  Constant1 : Constant  Value=0
  Constant2 : Constant  Value=delta_t
  Constant3 : Constant  Value=0
  Cross Product : matrix_library/Cross Product
  Degrees to Radians : simulink_extras/Transformations/Degrees to Radians
  Delay : Delay  DelayLength=1
  Demux : Demux  Outputs=3
  Discrete Derivative : simulink/Discrete/Discrete Derivative  Commented=on  gainval=1.0  ICPrevScaledInput=0.0  OutMin=[]  OutMax=[]  OutDataType=fixdt(1, 16)  OutScaling=2^-10  DoSatur=off
  Gain : Gain  Gain=k_p_mahony
  Gain1 : Gain  Gain=k_i_mahony
  Gain2 : Gain  Gain=delta_t
  Gyro - Bias - Removal : Subsystem  Commented=on
  Lowpass Filter : dspfdesign/Lowpass Filter  FilterType=FIR  DesignForMinimumOrder=on  FilterOrder=50  PassbandFrequency=0.0005  StopbandFrequency=0.002442  PassbandRipple=0.1  StopbandAttenuation=80  SampleRateMode=Use normalized frequency (0 to 1)  SampleRate=44100  SimulateUsing=Interpreted execution  roundingMode=Floor  coeffsDataTypeStr=fixdt(1,16)
  MATLAB Function : MATLAB Function  TreatAsAtomicUnit=on
  MATLAB Function1 : MATLAB Function  TreatAsAtomicUnit=on  SystemSampleTime=delta_t
  MATLAB Function2 : MATLAB Function  TreatAsAtomicUnit=on
  Mux : Mux  Inputs=3
  Sample and Hold : dspsigops/Sample and Hold  trig=Rising edge  initCond=0  latchinput=off
  Scope1 : Scope
  Selector : Selector  InputPortWidth=3  IndexOptions=Index vector (dialog)  Indices=[3]  OutputSizes=1
  Selector1 : Selector  InputPortWidth=2  IndexOptions=Index vector (dialog)  Indices=[2]  OutputSizes=1
  Selector2 : Selector  InputPortWidth=3  IndexOptions=Index vector (dialog)  Indices=[3]  OutputSizes=1
  Step : Step  Time=step_time  SampleTime=delta_t
  Step1 : Step  Commented=on  Time=step_time  SampleTime=delta_t
  Step2 : Step  Time=step_time  SampleTime=delta_t
  Sum : Sum  Inputs=++|
  Sum1 : Sum  Inputs=|++|
  Sum2 : Sum  Inputs=|+-
  Sum5 : Sum  Inputs=|++
  Switch : Switch  Threshold=0.1  SaturateOnIntegerOverflow=off  InputSameDT=off
  Switch1 : Switch  Threshold=1  SaturateOnIntegerOverflow=off  InputSameDT=off
  Unit Delay : UnitDelay  InitialCondition=q_init  SampleTime=delta_t  HasFrameUpgradeWarning=on
  Unit Delay1 : UnitDelay  SampleTime=-1  HasFrameUpgradeWarning=on
  Unit Delay3 : UnitDelay  SampleTime=delta_t  HasFrameUpgradeWarning=on
  lowpassed_raw_yaw : Scope
  normalize_g_b : MATLAB Function  TreatAsAtomicUnit=on
  euler : Outport
  Bias : Outport  Port=2
  wires:
  MATLAB Function1/1(euler) -> euler/1, Selector/1
  Accel/1 -> normalize_g_b/1(g_b)  "g_b"
  Gyro/1 -> Degrees to Radians/1  "omega"
  Sum1/1 -> Scope1/1, Sum/2  "delta_omega"
  Constant/1 -> MATLAB Function1/2(delta_t)
  Degrees to Radians/1 -> Demux/1  "original"
  MATLAB Function2/1(v_b) -> Cross Product/2
  Gain/1 -> Sum1/1
  Gain1/1 -> Gain2/1
  Cross Product/1 -> Gain1/1, Gain/1
  Unit Delay3/1 -> Sum1/2, Sum5/2
  Sum/1 -> MATLAB Function1/1(omega)
  normalize_g_b/1(g_b_norm) -> Cross Product/1
  Unit Delay/1 -> MATLAB Function2/1(q), MATLAB Function1/3(quat_mem)
  MATLAB Function1/2(quaternion_tplus) -> Unit Delay/1
  Gain2/1 -> Sum5/1
  Sum5/1 -> Unit Delay3/1
  Selector/1 -> BIAS-ESO/2(Yaw_Fused)
  Constant1/1 -> Switch/3
  BIAS-ESO/1(Bias) -> Bias/1, Selector1/1
  Step/1 -> Sample and Hold/Trigger
  Selector1/1 -> Unit Delay1/1
  Demux/3 -> Sum2/1
  Sum2/1 -> Mux/3
  Mux/1 -> Sum/1
  Demux/2 -> Mux/2
  Demux/1 -> Mux/1
  Unit Delay1/1 -> Switch1/1
  Sample and Hold/1 -> Sum2/2
  Step1/1 -> ?
  rpy/1 -> Selector2/1
  Lowpass Filter/1 -> lowpassed_raw_yaw/1, MATLAB Function/1(yaw_est), Delay/1
  Delay/1 -> MATLAB Function/2(prev_yaw_est)
  Constant2/1 -> MATLAB Function/3(delta_t)
  MATLAB Function/1(omega_yaw_est) -> Switch/1, Switch/2
  Switch/1 -> BIAS-ESO/1(u)
  Constant3/1 -> Switch1/3
  Step2/1 -> Switch1/2
  Switch1/1 -> BiasEst/1, Sample and Hold/1
  Selector2/1 -> Lowpass Filter/1

== system AttitudePlayground/P3022-V1- CW360 -Interface ==
  Analog Input : bbblueBasicLib/Analog Input  Pin=AIN0  Mode=Volt  SampleTime=delta_t  SimulateUsing=Code generation
  Display : Display
  Gain : Gain  Gain=-1/voltage_divider_Vout_max
  Gain1 : Gain  Gain=360
  Gain2 : Gain  Gain=2*pi
  Yaw (Rad) : Outport
  Yaw (Deg) : Outport  Port=2
  wires:
  Gain/1 -> Gain2/1, Gain1/1
  Analog Input/1 -> Display/1, Gain/1
  Gain2/1 -> Yaw (Rad)/1  "Yaw (Rad)"
  Gain1/1 -> Yaw (Deg)/1  "Yaw (Deg)"

== system AttitudePlayground/Quarternion EKF ==
  Accel : Inport
  Mag : Inport  Port=2
  Gyro : Inport  Port=3
  q_init : Inport  Port=4
  Constant : Constant  Value=delta_t
  Constant1 : Constant  Value=gyro_sigma
  Constant2 : Constant  Value=r_qekf
  Constant3 : Constant  Value=acc_sigma
  Constant4 : Constant  Value=mag_sigma
  Degrees to Radians : simulink_extras/Transformations/Degrees to Radians
  Delay : Delay  DelayLength=1  InitialConditionSource=Input port  SampleTime=delta_t
      settings: InputPortMap=u0,p4
  MATLAB Function : MATLAB Function  TreatAsAtomicUnit=on
  Predict : MATLAB Function  TreatAsAtomicUnit=on
  Unit Delay1 : UnitDelay  InitialCondition=P_0  SampleTime=delta_t  HasFrameUpgradeWarning=on
  Update : MATLAB Function  TreatAsAtomicUnit=on  SystemSampleTime=delta_t
  normalize_g_b : MATLAB Function  TreatAsAtomicUnit=on
  normalize_vec : MATLAB Function  TreatAsAtomicUnit=on
  q : Outport
  euler_qekf : Outport  Port=2
  wires:
  Update/1(q_t) -> Delay/1, q/1, MATLAB Function/1(quat_in)  "outputs"
  Accel/1 -> normalize_g_b/1(v)
  Mag/1 -> normalize_vec/1(v)
  Constant/1 -> Predict/3(delta_t)
  Unit Delay1/1 -> Predict/4(P_t_)
  Update/2(P_t) -> Unit Delay1/1
  Predict/1(q_t_dash) -> Update/3(quat_in)
  normalize_g_b/1(v_norm) -> Update/1(accel)
  normalize_vec/1(v_norm) -> Update/2(mag)
  Constant2/1 -> Update/4(r)
  Constant3/1 -> Update/5(acc_sigma)
  Constant4/1 -> Update/6(mag_sigma)
  Delay/1 -> Predict/1(quat_in)
  Predict/2(P_t_dash) -> Update/7(P_t_dash)
  MATLAB Function/1(euler) -> euler_qekf/1
  Degrees to Radians/1 -> Predict/2(omega)  "u"
  Gyro/1 -> Degrees to Radians/1  "original"
  Constant1/1 -> Predict/5(gyro_sigma)
  q_init/1 -> Delay/2

== system AttitudePlayground/Quarternion EKF + Amfitrack ==
  Accel : Inport
  Gyro : Inport  Port=2
  q_amfitrack : Inport  Port=3
  Constant : Constant  Value=delta_t
  Constant1 : Constant  Value=gyro_sigma_3d
  Constant2 : Constant  Value=q_sigma
  Constant3 : Constant  Value=acc_sigma
  Degrees to Radians : simulink_extras/Transformations/Degrees to Radians
  Delay : Delay  DelayLength=1  InitialCondition=[1,0,0,0]  SampleTime=delta_t
  MATLAB Function : MATLAB Function  TreatAsAtomicUnit=on
  Predict : MATLAB Function  TreatAsAtomicUnit=on
  Unit Delay1 : UnitDelay  InitialCondition=P_0  SampleTime=delta_t  HasFrameUpgradeWarning=on
  Update : MATLAB Function  TreatAsAtomicUnit=on  SystemSampleTime=delta_t
  normalize_g_b : MATLAB Function  TreatAsAtomicUnit=on
  q : Outport
  euler_qekf : Outport  Port=2
  wires:
  Update/1(q_t) -> Delay/1, q/1, MATLAB Function/1(quat_in)  "outputs"
  Accel/1 -> normalize_g_b/1(v)
  Constant/1 -> Predict/3(delta_t)
  Unit Delay1/1 -> Predict/4(P_t_)
  Update/2(P_t) -> Unit Delay1/1
  Predict/1(q_t_dash) -> Update/3(quat_in)
  normalize_g_b/1(v_norm) -> Update/1(accel)
  Constant3/1 -> Update/4(acc_sigma)
  Delay/1 -> Predict/1(quat_in)
  Predict/2(P_t_dash) -> Update/6(P_t_dash)
  MATLAB Function/1(euler) -> euler_qekf/1
  Degrees to Radians/1 -> Predict/2(omega)  "u"
  Gyro/1 -> Degrees to Radians/1  "original"
  Constant1/1 -> Predict/5(gyro_sigma)
  q_amfitrack/1 -> Update/2(q_meas)
  Constant2/1 -> Update/5(q_sigma)

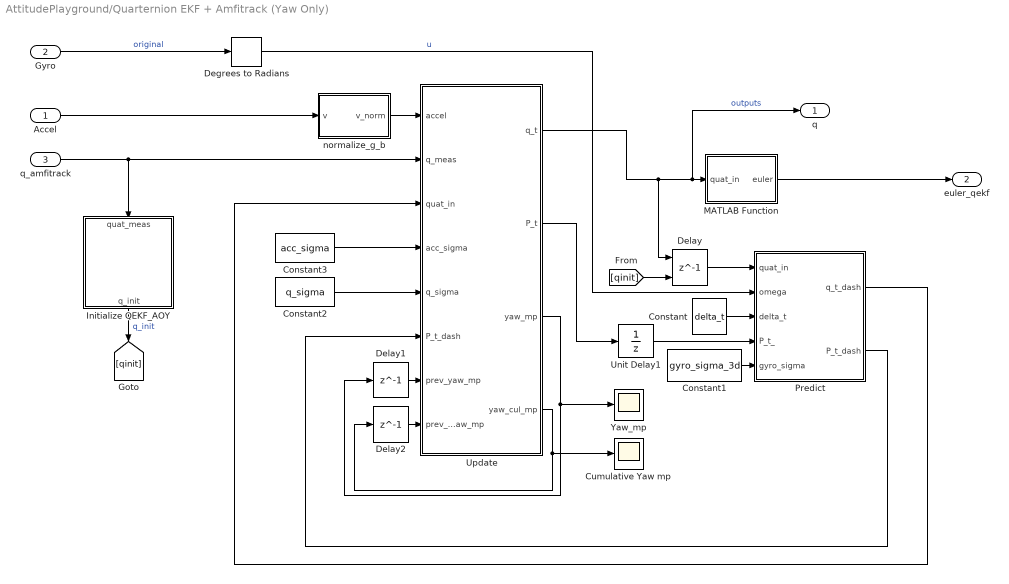
== system AttitudePlayground/Quarternion EKF + Amfitrack (Yaw Only) ==
  Accel : Inport
  Gyro : Inport  Port=2
  q_amfitrack : Inport  Port=3
  Constant : Constant  Value=delta_t
  Constant1 : Constant  Value=gyro_sigma_3d
  Constant2 : Constant  Value=q_sigma
  Constant3 : Constant  Value=acc_sigma
  Cumulative Yaw mp : Scope
  Degrees to Radians : simulink_extras/Transformations/Degrees to Radians
  Delay : Delay  DelayLength=1  InitialConditionSource=Input port  InitialCondition=[1,0,0,0]  SampleTime=delta_t
      settings: InputPortMap=u0,p4
  Delay1 : Delay  DelayLength=1  InitialCondition=[0,0]  SampleTime=delta_t
  Delay2 : Delay  DelayLength=1  InitialCondition=[0,0]  SampleTime=delta_t
  Initialize QEKF_AOY : MATLAB Function  TreatAsAtomicUnit=on
  MATLAB Function : MATLAB Function  TreatAsAtomicUnit=on
  Predict : MATLAB Function  TreatAsAtomicUnit=on
  Unit Delay1 : UnitDelay  InitialCondition=P_0  SampleTime=delta_t  HasFrameUpgradeWarning=on
  Update : MATLAB Function  TreatAsAtomicUnit=on  SystemSampleTime=delta_t
  Yaw_mp : Scope
  normalize_g_b : MATLAB Function  TreatAsAtomicUnit=on
  q : Outport
  euler_qekf : Outport  Port=2
  wires:
  Update/1(q_t) -> Delay/1, q/1, MATLAB Function/1(quat_in)  "outputs"
  Accel/1 -> normalize_g_b/1(v)
  Constant/1 -> Predict/3(delta_t)
  Unit Delay1/1 -> Predict/4(P_t_)
  Update/2(P_t) -> Unit Delay1/1
  Predict/1(q_t_dash) -> Update/3(quat_in)
  normalize_g_b/1(v_norm) -> Update/1(accel)
  Constant3/1 -> Update/4(acc_sigma)
  Delay/1 -> Predict/1(quat_in)
  Predict/2(P_t_dash) -> Update/6(P_t_dash)
  MATLAB Function/1(euler) -> euler_qekf/1
  Degrees to Radians/1 -> Predict/2(omega)  "u"
  Gyro/1 -> Degrees to Radians/1  "original"
  Constant1/1 -> Predict/5(gyro_sigma)
  q_amfitrack/1 -> Update/2(q_meas), Initialize QEKF_AOY/1(quat_meas)
  Constant2/1 -> Update/5(q_sigma)
  Delay1/1 -> Update/7(prev_yaw_mp)
  Delay2/1 -> Update/8(prev_cul_yaw_mp)
  Update/3(yaw_mp) -> Delay1/1, Yaw_mp/1
  Update/4(yaw_cul_mp) -> Delay2/1, Cumulative Yaw mp/1
  Initialize QEKF_AOY/1(q_init) -> [qinit]  "q_init"
  [qinit] -> Delay/2

== system AttitudePlayground/Quarternion EKF + Amfitrack (Yaw Only)1 ==
  Accel : Inport
  Gyro : Inport  Port=2
  q_amfitrack : Inport  Port=3
  Constant : Constant  Value=delta_t
  Constant1 : Constant  Value=gyro_sigma_3d
  Constant2 : Constant  Value=q_sigma
  Constant3 : Constant  Value=acc_sigma
  Cumulative Yaw mp : Scope
  Degrees to Radians : simulink_extras/Transformations/Degrees to Radians
  Delay : Delay  DelayLength=1  InitialCondition=[1,0,0,0]  SampleTime=delta_t
  Delay1 : Delay  DelayLength=1  InitialCondition=[0,0]  SampleTime=delta_t
  Delay2 : Delay  DelayLength=1  InitialCondition=[0,0]  SampleTime=delta_t
  MATLAB Function : MATLAB Function  TreatAsAtomicUnit=on
  Predict : MATLAB Function  TreatAsAtomicUnit=on
  Unit Delay1 : UnitDelay  InitialCondition=P_0  SampleTime=delta_t  HasFrameUpgradeWarning=on
  Update : MATLAB Function  TreatAsAtomicUnit=on  SystemSampleTime=delta_t
  Yaw_mp : Scope
  normalize_g_b : MATLAB Function  TreatAsAtomicUnit=on
  q : Outport
  euler_qekf : Outport  Port=2
  wires:
  Update/1(q_t) -> Delay/1, q/1, MATLAB Function/1(quat_in)  "outputs"
  Accel/1 -> normalize_g_b/1(v)
  Constant/1 -> Predict/3(delta_t)
  Unit Delay1/1 -> Predict/4(P_t_)
  Update/2(P_t) -> Unit Delay1/1
  Predict/1(q_t_dash) -> Update/3(quat_in)
  normalize_g_b/1(v_norm) -> Update/1(accel)
  Constant3/1 -> Update/4(acc_sigma)
  Delay/1 -> Predict/1(quat_in)
  Predict/2(P_t_dash) -> Update/6(P_t_dash)
  MATLAB Function/1(euler) -> euler_qekf/1
  Degrees to Radians/1 -> Predict/2(omega)  "u"
  Gyro/1 -> Degrees to Radians/1  "original"
  Constant1/1 -> Predict/5(gyro_sigma)
  q_amfitrack/1 -> Update/2(q_meas)
  Constant2/1 -> Update/5(q_sigma)
  Delay1/1 -> Update/7(prev_yaw_mp)
  Delay2/1 -> Update/8(prev_cul_yaw_mp)
  Update/3(yaw_mp) -> Delay1/1, Yaw_mp/1
  Update/4(yaw_cul_mp) -> Delay2/1, Cumulative Yaw mp/1

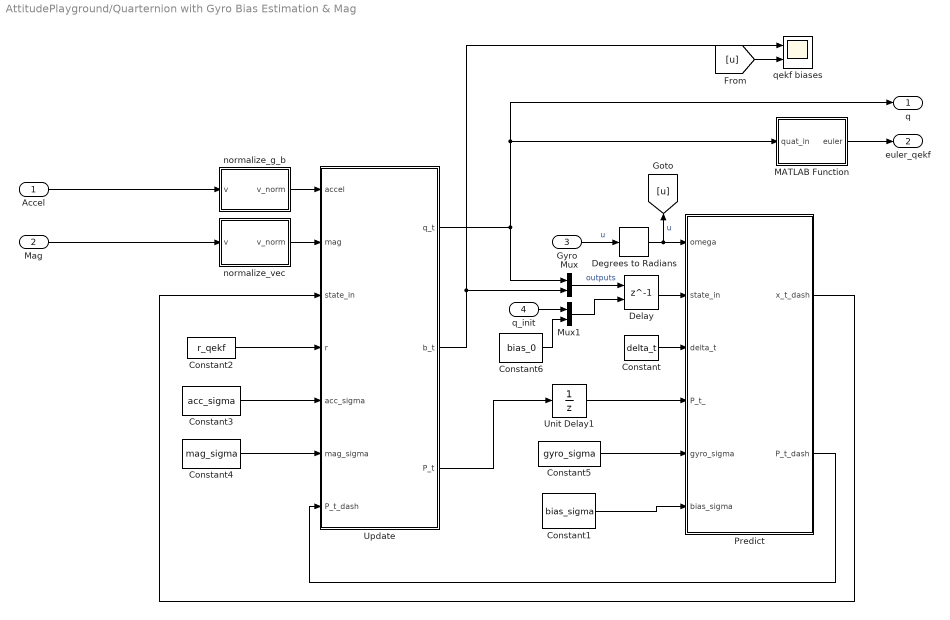
== system AttitudePlayground/Quarternion with Gyro Bias Estimation & Mag ==
  Accel : Inport
  Mag : Inport  Port=2
  Gyro : Inport  Port=3
  q_init : Inport  Port=4
  Constant : Constant  Value=delta_t
  Constant1 : Constant  Value=bias_sigma
  Constant2 : Constant  Value=r_qekf
  Constant3 : Constant  Value=acc_sigma
  Constant4 : Constant  Value=mag_sigma
  Constant5 : Constant  Value=gyro_sigma
  Constant6 : Constant  Value=bias_0
  Degrees to Radians : simulink_extras/Transformations/Degrees to Radians
  Delay : Delay  DelayLength=1  InitialConditionSource=Input port  SampleTime=delta_t
      settings: InputPortMap=u0,p4
  MATLAB Function : MATLAB Function  TreatAsAtomicUnit=on
  Mux : Mux  Inputs=2
  Mux1 : Mux  Inputs=2
  Predict : MATLAB Function  TreatAsAtomicUnit=on
  Unit Delay1 : UnitDelay  InitialCondition=P_0_gb  SampleTime=delta_t  HasFrameUpgradeWarning=on
  Update : MATLAB Function  TreatAsAtomicUnit=on  SystemSampleTime=delta_t
  normalize_g_b : MATLAB Function  TreatAsAtomicUnit=on
  normalize_vec : MATLAB Function  TreatAsAtomicUnit=on
  qekf biases : Scope  NumInputPorts=2
  q : Outport
  euler_qekf : Outport  Port=2
  wires:
  Update/1(q_t) -> MATLAB Function/1(quat_in), q/1, Mux/1
  Accel/1 -> normalize_g_b/1(v)
  Mag/1 -> normalize_vec/1(v)
  Constant/1 -> Predict/3(delta_t)
  Unit Delay1/1 -> Predict/4(P_t_)
  Update/3(P_t) -> Unit Delay1/1
  Predict/1(x_t_dash) -> Update/3(state_in)
  normalize_g_b/1(v_norm) -> Update/1(accel)
  normalize_vec/1(v_norm) -> Update/2(mag)
  Constant2/1 -> Update/4(r)
  Constant3/1 -> Update/5(acc_sigma)
  Constant4/1 -> Update/6(mag_sigma)
  Delay/1 -> Predict/2(state_in)
  Predict/2(P_t_dash) -> Update/7(P_t_dash)
  Gyro/1 -> Degrees to Radians/1  "u"
  MATLAB Function/1(euler) -> euler_qekf/1
  Degrees to Radians/1 -> [u], Predict/1(omega)  "u"
  Constant1/1 -> Predict/6(bias_sigma)
  Constant5/1 -> Predict/5(gyro_sigma)
  Update/2(b_t) -> qekf biases/1, Mux/2
  Mux/1 -> Delay/1  "outputs"
  q_init/1 -> Mux1/1
  Mux1/1 -> Delay/2
  Constant6/1 -> Mux1/2
  [u] -> qekf biases/2

== system AttitudePlayground/Quarternion with Gyro Bias Estimation & no Mag ==
  Accel : Inport
  Gyro : Inport  Port=2
  Constant : Constant  Value=delta_t
  Constant1 : Constant  Value=bias_sigma
  Constant3 : Constant  Value=acc_sigma
  Constant5 : Constant  Value=gyro_sigma
  Degrees to Radians : simulink_extras/Transformations/Degrees to Radians
  MATLAB Function : MATLAB Function  TreatAsAtomicUnit=on
  Mux : Mux  Inputs=2
  Predict : MATLAB Function  TreatAsAtomicUnit=on
  Unit Delay : UnitDelay  InitialCondition=[q_init bias_0]  SampleTime=delta_t  HasFrameUpgradeWarning=on
  Unit Delay1 : UnitDelay  InitialCondition=P_0_gb  SampleTime=delta_t  HasFrameUpgradeWarning=on
  Update : MATLAB Function  TreatAsAtomicUnit=on  SystemSampleTime=delta_t
  normalize_g_b : MATLAB Function  TreatAsAtomicUnit=on
  qekf biases : Scope
  q : Outport
  euler_qekf : Outport  Port=2
  wires:
  Update/1(q_t) -> q/1, MATLAB Function/1(quat_in), Mux/1
  Accel/1 -> normalize_g_b/1(v)
  Constant/1 -> Predict/3(delta_t)
  Unit Delay1/1 -> Predict/4(P_t_)
  Update/3(P_t) -> Unit Delay1/1
  Predict/1(x_t_dash) -> Update/2(state_in)
  normalize_g_b/1(v_norm) -> Update/1(accel)
  Constant3/1 -> Update/3(acc_sigma)
  Unit Delay/1 -> Predict/1(state_in)
  Predict/2(P_t_dash) -> Update/4(P_t_dash)
  Gyro/1 -> Degrees to Radians/1  "u"
  MATLAB Function/1(euler) -> euler_qekf/1
  Degrees to Radians/1 -> Predict/2(omega)  "u"
  Constant1/1 -> Predict/6(bias_sigma)
  Constant5/1 -> Predict/5(gyro_sigma)
  Update/2(b_t) -> qekf biases/1, Mux/2
  Mux/1 -> Unit Delay/1

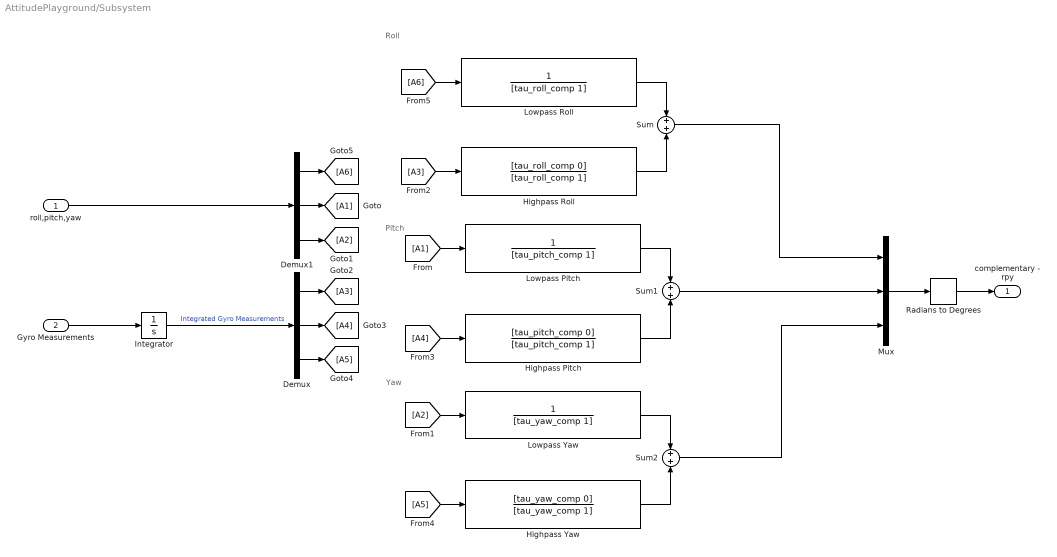
== system AttitudePlayground/Subsystem ==
  note: Yaw
  note: Pitch
  note: Roll
  roll,pitch,yaw : Inport
  Gyro Measurements : Inport  Port=2
  Demux : Demux  Outputs=3
  Demux1 : Demux  Outputs=3
  Highpass Pitch : TransferFcn  Numerator=[tau_pitch_comp 0]  Denominator=[tau_pitch_comp 1]
  "Highpass Roll " : TransferFcn  Numerator=[tau_roll_comp 0]  Denominator=[tau_roll_comp 1]
  Highpass Yaw : TransferFcn  Numerator=[tau_yaw_comp 0]  Denominator=[tau_yaw_comp 1]
  Integrator : Integrator
  Lowpass Pitch : TransferFcn  Denominator=[tau_pitch_comp 1]
  Lowpass Roll : TransferFcn  Denominator=[tau_roll_comp 1]
  Lowpass Yaw : TransferFcn  Denominator=[tau_yaw_comp 1]
  Mux : Mux  Inputs=3
  Radians to Degrees : simulink_extras/Transformations/Radians to Degrees
  Sum : Sum
  Sum1 : Sum
  Sum2 : Sum
  complementary - rpy : Outport
  wires:
  Gyro Measurements/1 -> Integrator/1
  "Highpass Roll "/1 -> Sum/2
  Integrator/1 -> Demux/1  "Integrated Gyro Measurements"
  roll,pitch,yaw/1 -> Demux1/1
  Lowpass Roll/1 -> Sum/1
  Mux/1 -> Radians to Degrees/1
  Sum/1 -> Mux/1
  Highpass Pitch/1 -> Sum1/2
  Lowpass Pitch/1 -> Sum1/1
  Sum1/1 -> Mux/2
  Sum2/1 -> Mux/3
  Highpass Yaw/1 -> Sum2/2
  Lowpass Yaw/1 -> Sum2/1
  Radians to Degrees/1 -> complementary - rpy/1
  Demux1/2 -> [A1]
  [A1] -> Lowpass Pitch/1
  Demux1/3 -> [A2]
  [A2] -> Lowpass Yaw/1
  Demux/1 -> [A3]
  [A3] -> "Highpass Roll "/1
  Demux/2 -> [A4]
  [A4] -> Highpass Pitch/1
  Demux/3 -> [A5]
  [A5] -> Highpass Yaw/1
  Demux1/1 -> [A6]
  [A6] -> Lowpass Roll/1
